simulink model "gastank1"  (R2018b)
settings: Solver=ode45  StartTime=0.0  StopTime=8640  RelTol=1e-3
values from neighbouring files (symbols this model uses):
  A = 1    [gastank.m]    (also in tank.m = 3)
  a2 = 5*exp(-4)    [gastank.m]
  g = 9.81    [gastank.m]    (also in tank.m)
  pG = 3*exp(5)    [gastank.m]
  pL = 1*exp(5)    [gastank.m]
  pzu = 8.943*exp(5)    [gastank.m]
  qzu = 5    [gastank.m]    (also in tank.m)
  rho = 1000    [gastank.m]
settings Model: Creator=Naveen  LastModifiedBy=Naveen

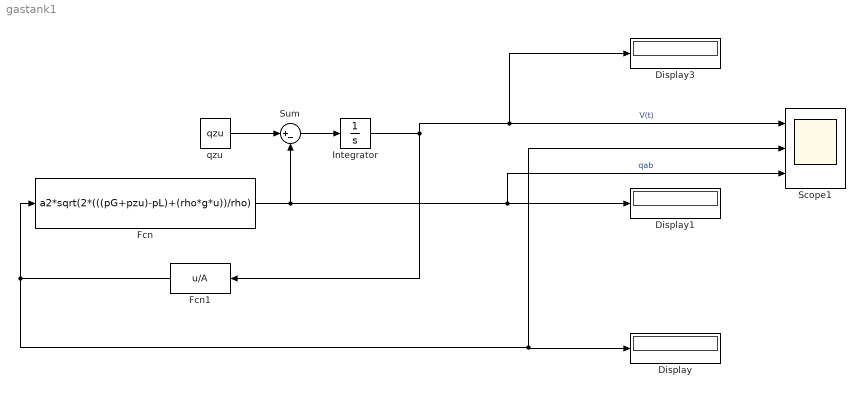
== system gastank1 ==
  Display : Display
  Display1 : Display
  Display3 : Display
  Fcn : Fcn  Expr=a2*sqrt(2*(((pG+pzu)-pL)+(rho*g*u))/rho)
  Fcn1 : Fcn  Expr=u/A
  Integrator : Integrator
  Scope1 : Scope  NumInputPorts=3
  Sum : Sum  Inputs=|+-
  qzu : Constant  Value=qzu
  wires:
  Fcn1/1 -> Display/1, Scope1/2, Fcn/1
  Integrator/1 -> Fcn1/1, Scope1/1, Display3/1  "V(t)"
  Sum/1 -> Integrator/1
  Fcn/1 -> Sum/2, Scope1/3, Display1/1  "qab"
  qzu/1 -> Sum/1
